simulink model "therm_model"  (Simulink 7.5)
settings: Solver=ode45  StartTime=0.0  StopTime=48  RelTol=1e-3  AbsTol=1e-6
values from neighbouring files (symbols this model uses):
  c = 1005.4    [househeat_data.m]    (also in thermSim.m)
  M = (lenHouse*widHouse*htHouse+tan(pitRoof)*widHouse*lenHouse)*densAir    [househeat_data.m]    (also in thermSim.m)
  Mdot = 3600    [househeat_data.m]    (also in thermSim.m)
  Req = RWall*RWindow/(RWall + RWindow)    [househeat_data.m]    (also in thermSim.m = Req * Req_sf)
  THeater = 50    [househeat_data.m]    (also in thermSim.m = THeater * THeater_sf)
  TinIC = (70-32)*5/9    (= 21.1111111111)    [househeat_data.m]    (also in thermSim.m)
settings Model: Creator=gregfiore  LastModifiedBy=gregfiore

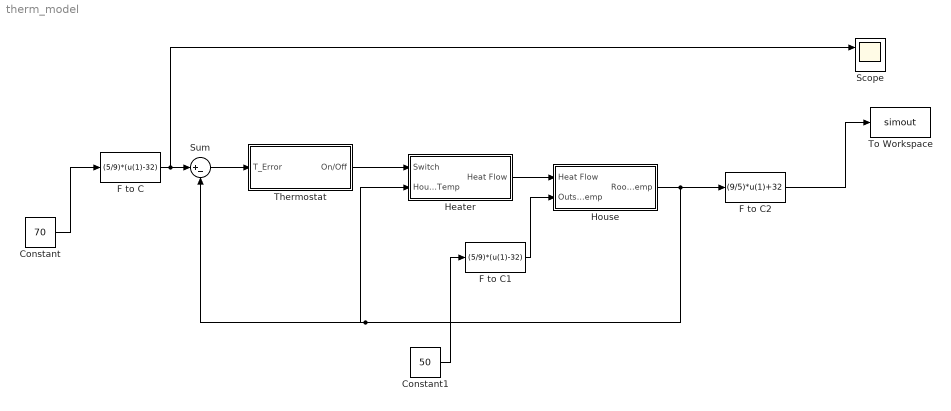
== system therm_model ==
  Constant : Constant  Value=70  OutDataType=fixdt(1, 16)  OutScaling=2^0
  Constant1 : Constant  Value=50  OutDataType=fixdt(1, 16)  OutScaling=2^0
  F to C : Fcn  Expr=(5/9)*(u(1)-32)
  F to C1 : Fcn  Expr=(5/9)*(u(1)-32)
  F to C2 : Fcn  Expr=(9/5)*u(1)+32
  Heater : Subsystem
  House : Subsystem
  Scope : Scope  NumInputPorts=2
      settings: YMin=-5~-5  YMax=5~5
  Sum : Sum  Inputs=|+-  OutDataType=fixdt(1, 16)  OutScaling=2^0
  Thermostat : Subsystem
  To Workspace : ToWorkspace  VariableName=simout  SampleTime=-1  SaveFormat=Structure
  wires:
  Thermostat/1(On/Off) -> Heater/1(Switch)
  Heater/1(Heat Flow) -> House/1(Heat Flow)
  House/1(Room Temp) -> Sum/2, Heater/2(House Temp), F to C2/1
  Sum/1 -> Thermostat/1(T_Error)
  F to C/1 -> Sum/1, Scope/1
  F to C1/1 -> House/2(Outside Temp)
  F to C2/1 -> To Workspace/1
  Constant/1 -> F to C/1
  Constant1/1 -> F to C1/1

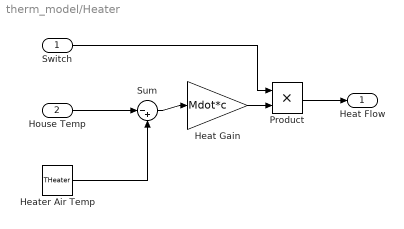
== system therm_model/Heater ==
  Switch : Inport  OutDataType=fixdt(1, 16)  OutScaling=2^0
  House Temp : Inport  Port=2  OutDataType=fixdt(1, 16)  OutScaling=2^0
  Heat Gain : Gain  Gain=Mdot*c  ParameterDataType=fixdt(1, 16)  ParameterScaling=2^0  OutDataType=fixdt(1, 16)  OutScaling=2^0
  Heater Air Temp : Constant  Value=THeater  OutDataType=fixdt(1, 16)  OutScaling=2^0
  Product : Product  OutDataType=fixdt(1, 16)  OutScaling=2^0  RndMeth=Zero
  Sum : Sum  Inputs=|-+  OutDataType=fixdt(1, 16)  OutScaling=2^0
  Heat Flow : Outport  OutDataType=fixdt(1, 16)  OutScaling=2^0
  wires:
  House Temp/1 -> Sum/1
  Heater Air Temp/1 -> Sum/2
  Sum/1 -> Heat Gain/1
  Heat Gain/1 -> Product/2
  Switch/1 -> Product/1
  Product/1 -> Heat Flow/1

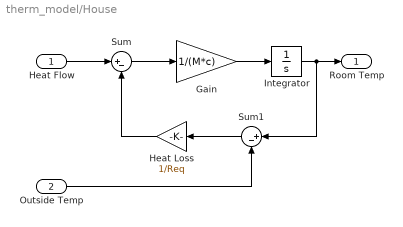
== system therm_model/House ==
  Heat Flow : Inport  OutDataType=fixdt(1, 16)  OutScaling=2^0
  Outside Temp : Inport  Port=2  OutDataType=fixdt(1, 16)  OutScaling=2^0
  Gain : Gain  Gain=1/(M*c)  ParameterDataType=fixdt(1, 16)  ParameterScaling=2^0  OutDataType=fixdt(1, 16)  OutScaling=2^0
  Heat Loss : Gain  Gain=1/Req  ParameterDataType=fixdt(1, 16)  ParameterScaling=2^0  OutDataType=fixdt(1, 16)  OutScaling=2^0
  Integrator : Integrator  InitialCondition=TinIC
  Sum : Sum  Inputs=|+-  OutDataType=fixdt(1, 16)  OutScaling=2^0
  Sum1 : Sum  Inputs=|+-  OutDataType=fixdt(1, 16)  OutScaling=2^0
  Room Temp : Outport  OutDataType=fixdt(1, 16)  OutScaling=2^0
  wires:
  Sum/1 -> Gain/1
  Heat Flow/1 -> Sum/1
  Integrator/1 -> Room Temp/1, Sum1/1
  Gain/1 -> Integrator/1
  Outside Temp/1 -> Sum1/2
  Sum1/1 -> Heat Loss/1
  Heat Loss/1 -> Sum/2

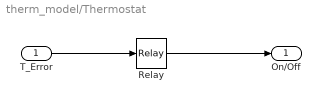
== system therm_model/Thermostat ==
  T_Error : Inport  OutDataType=fixdt(1, 16)  OutScaling=2^0
  Relay : Relay  OnSwitchValue=5*(5/9)  OffSwitchValue=-5*(5/9)  OutDataType=fixdt(1, 16)  OutScaling=2^0
  On/Off : Outport  OutDataType=fixdt(1, 16)  OutScaling=2^0
  wires:
  T_Error/1 -> Relay/1
  Relay/1 -> On/Off/1
